simulink model "Hybrid_car_model"  (R2023a)
settings: Solver=VariableStepAuto  StartTime=0.0  StopTime=7200  MaxStep=0.05  RelTol=1e-3
values from neighbouring files (symbols this model uses):
  Af = 0.6    [a_Vehicle_Data.m]
  Cd = 0.5    [a_Vehicle_Data.m]
  eta_dt = 0.95    [a_Vehicle_Data.m]
  fR = 0.020    (= 0.02)    [a_Vehicle_Data.m]
  g = 9.81    [a_Vehicle_Data.m]
  gamma = 0    [a_Vehicle_Data.m]
  i_1 = 31/12    (= 2.58333333333)    [a_Vehicle_Data.m]
  i_2 = 25/13    (= 1.92307692308)    [a_Vehicle_Data.m]
  i_3 = 23/15    (= 1.53333333333)    [a_Vehicle_Data.m]
  i_4 = 24/19    (= 1.26315789474)    [a_Vehicle_Data.m]
  i_fin = 36/13    (= 2.76923076923)    [a_Vehicle_Data.m]
  i_prim = 56/22    (= 2.54545454545)    [a_Vehicle_Data.m]
  K_e = 1/54    (= 0.0185185185185)    [c_electric_motor_data.m]
  K_t = 0.15    [c_electric_motor_data.m]
  L_a = 23e-6    (= 2.3e-05)    [c_electric_motor_data.m]
  m = 250    [a_Vehicle_Data.m]
  R_a = 22.5e-3    (= 0.0225)    [c_electric_motor_data.m]
  r_dyn = 0.227    [a_Vehicle_Data.m]
  rho = 1.225    [a_Vehicle_Data.m]
  time_demand = [0;1;2;3;4;5;6;7;8;9;10;11;12;13;14;15;16;17;18;19;20;21;22;23;24;25;26;27;28;29;30;31;32;33;34;35;36;37;38;39;40;41;42;43;44;45;46;47;48;49;50;51;52;53;54;55;56;57;58;59;60;61;62;63;64;65;66;67;68;69;70;71;72;73;74;75;76;77;78;79;80;81;82;83;84;85;86;87;88;89;90;91;92;93;94;95;96;97;98;99;100;101;102;103;104;105;106;107;108;109;110;111;112;113;114;115;116;117;118;119;120;121;122;123;124;125;126;1 ...(+7496 chars)    [WLTP_data.m]
  velocity_demand = [0;0;0;0;0;0;0;0;0;0;0;0;0.200000000000000;1.70000000000000;5.40000000000000;9.90000000000000;13.1000000000000;16.9000000000000;21.7000000000000;26;27.5000000000000;28.1000000000000;28.3000000000000;28.8000000000000;29.1000000000000;30.8000000000000;31.9000000000000;34.1000000000000;36.6000000000000;39.1000000000000;41.3000000000000;42.5000000000000;43.3000000000000;43.9000000000000;44.40000000000 ...(+24040 chars)    [WLTP_data.m]
undefined symbols (not defined in the file or in its folder): Hydride, Metal, Nickel
libraries: spsCurrentMeasurementLib x2, spsBatteryLib x1, spsControlledCurrentSourceLib x1, spsDCMachineLib x1, sps_lib x1, slpidlib x1
settings Model: Creator=jens.lahr  LastModifiedBy=id306071
settings ModelReferenceCC: EnableRefExpFcnMdlSchedulingChecks=on

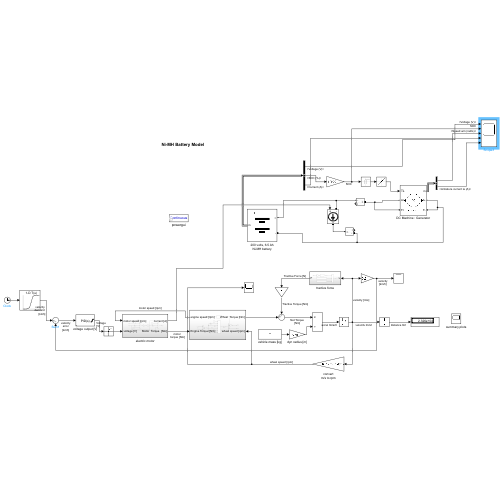
[thumbnail: Simulink's stored preview of the top-level diagram]
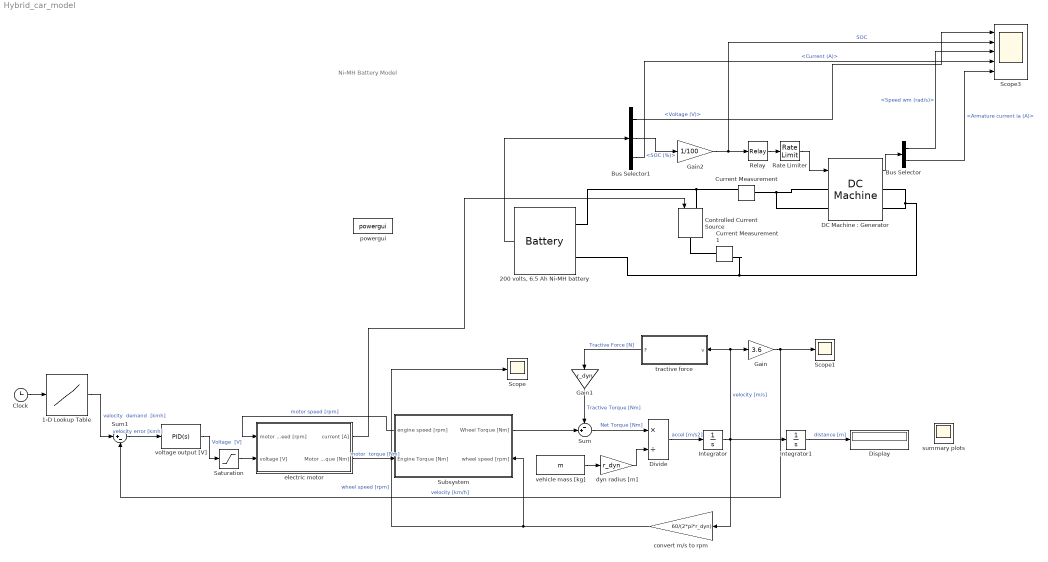
== system Hybrid_car_model ==
  note: Ni-MH Battery Model
  1-D Lookup Table : Lookup_n-D  NumberOfTableDimensions=1  BreakpointsForDimension1=time_demand  Table=velocity_demand  InternalRulePriority=Speed  RndMeth=Simplest
  "200 volts, 6.5 Ah Ni-MH battery " : spsBatteryLib/Battery  BatType=Nickel-Metal-Hydride  ShowTempParam=on  ThermalPreset=no  ShowAgeParam=off  NomV=200  NomQ=6.5  SOC=100  Batt_Tr=30  PresetModel=on  MaxQ=7  MinV=150  FullV=235.5932  Dis_rate=1.3  R=0.30769  Normal_OP=6.25  expZone="[216.9492           1.3]"  current=50  Units=Ampere-hour  Tci=20  NomT=25  T2=0  MaxQ2=2.208  FullV2=3.45  Normal_OP2=2.8  expZone2="[3.22        0.23]"  Rca=0.6  ti=1000  Dp=0  Neq0=0  Tsim=1e6  Ta1=25  Qeol=5.4*0.9  Reol=0.013333*1.2  Char_age=[2.3478, 3]  Dis_age=[2.3478, 10]  N1=1500  N2=10500  N3=1000  N4=1400  Ta2=45  N5=950
      settings: LibrarySourceBlock=electricdrivelib/Extra Sources/Battery
  Bus Selector : BusSelector  OutputSignals=Speed wm (rad/s),Armature current ia (A)
  Bus Selector1 : BusSelector  OutputSignals=Voltage (V),SOC (%),Current (A)
  Clock : Clock
  Controlled Current Source : spsControlledCurrentSourceLib/Controlled Current Source  Initialize=on  Source_Type=AC  Amplitude=0  Phase=0  Frequency=0  Measurements=None
  Current Measurement : spsCurrentMeasurementLib/Current Measurement  PhasorSimulation=off  OutputType=Complex  PSBequivalent=0
  Current Measurement1 : spsCurrentMeasurementLib/Current Measurement  PhasorSimulation=off  OutputType=Complex  PSBequivalent=0
  "DC Machine : Generator" : spsDCMachineLib/DC Machine  PresetModel=No  MechanicalLoad=Torque TL  FieldType=Wound  ShowDetailedParameters=on  MeasurementBus=off  RLa=[0.4832 0.006763]  RLf=[84.91 13.39]  Laf=0.7096  MachineConstant=Torque constant (N.m/A)  Ke=1.8  Kt=1.8  J=0.2053  Bm=0.007032  Tf=0  w0=0  Ifinit=0  TsPowergui=0  TsBlock=-1
  Display : Display
  Divide : Product  Inputs=*/
  Gain : Gain  Gain=3.6
  Gain1 : Gain  Gain=r_dyn
  Gain2 : Gain  Gain=1/100
  Integrator : Integrator  LimitOutput=on  LowerSaturationLimit=0
  Integrator1 : Integrator
  Rate Limiter : RateLimiter  RisingSlewLimit=100  FallingSlewLimit=-100
  Relay : Relay  OnSwitchValue=0.95  OffSwitchValue=0.2  OnOutputValue=0  OffOutputValue=-200
  Saturation : Saturate  UpperLimit=48  LowerLimit=0
  Scope : Scope
  Scope1 : Scope
  Scope3 : Scope  NumInputPorts=5
  Subsystem : Subsystem
      settings: PortSchema="{\"entries\":[{\"content\":{\"sides\":[{\"content\":{\"connectorIds\":[\"Out2\",\"In1\"]},\"type\":\"ConnectorPlacement.EquallySpacedRectSide\",\"uuid\":\"3db7130f-4414-4138-a483-769651bc2e03\"},{\"content\":{\"connectorIds\":[\"Out1\",\"In2\"],\"side\":\"RIGHT\"},\"type\":\"ConnectorPlacement.EquallySpacedRectSide\",\"uuid\":\"89f2a1b6-eda5-4fe5-b7f3-89dce8f6cd7c\"},{\"content\":{\"connectorIds\":[],\"side\":\"TOP\"},\"type\":\"ConnectorPlacement.EquallySpacedRectSide\",\"uuid\":\"e9ab6c0b-b883-402a-b7db-f259101e283a\"}]},\"type\":\"ConnectorPlacement.EquallySpacedConnector\",\"uuid\":\"5847757e-1c33-4a70-baac-f92835d7beeb\"}],\"packageUris\":[\"http://schema.mathworks.com/mf0/Connector/R2020b\"],\"version\":\"1.0\"}"
  Sum : Sum  Inputs=-+|
  Sum1 : Sum  Inputs=|+-
  convert m/s to rpm : Gain  Gain=60/(2*pi*r_dyn)
  dyn radius [m] : Gain  Gain=r_dyn
  electric motor : Subsystem
  powergui : sps_lib/powergui  SimulationMode=Continuous  SampleTime=0.001  frequency=60  Iterations=50  frequencyindice=0  Pbase=100e6  ErrMax=1e-4  UnitsV=kV  UnitsW=MW  buscounter=0  FunctionMessages=off  echomessages=off  EnableUseOfTLC=off  CurrentSourceSwitches=off  DisableSnubberDevices=off  DisableRonSwitches=off  DisableVfSwitches=off  DisplayEquations=off  AutomaticDiscreteSolvers=off  SolverType=Tustin  Interpol=off  ExternalGateDelay=off  methode=off  Ts=0  x0status=blocks  SPID=off  SwTol=0  HookPort=off  NonlinearTolerance=1e-4  nMaxIteration=100  ContinueOnMaxIteration=off  RestoreLinks=warning  ResistiveCurrentMeasurement=off  Frange=[0:2:500]  Ylog=off  Xlog=on  ShowGrid=off  save=off  variable=ZData  structure=0  ZoomFFT=on  StartTime=0.0  cycles=1  DisplayStyle=1  fundamental=60  FreqAxis=off  MaxFrequency=1000  frequencyindicesteady=1  RmsSteady=1  display=off
  summary plots : Scope
      settings: Floating=on
  tractive force : Subsystem
  vehicle mass [kg] : Constant  Value=m
  voltage output [V] : slpidlib/PID Controller  Controller=PID  Form=Parallel  TimeDomain=Continuous-time  UseExternalTs=off  SampleTime=-1  IntegratorMethod=Forward Euler  FilterMethod=Forward Euler  ControllerParametersSource=internal  P=23.06  I=0.5  UseKiTs=off  D=0  N=100  UseFilter=on  TunerSelectOption=Transfer Function Based (PID Tuner App)  InitialConditionSource=internal  InitialConditionForIntegrator=0  InitialConditionForFilter=0  DifferentiatorICPrevScaledInput=0  ExternalReset=none  TrackingMode=off  Kt=1  LimitOutput=on  SatLimitsSource=internal  UpperSaturationLimit=48  LowerSaturationLimit=0  LinearizeAsGain=on  AntiWindupMode=none  Kb=1  LimitIntegrator=off  UpperIntegratorSaturationLimit=inf  LowerIntegratorSaturationLimit=-inf  POutMin=[]  POutMax=[]  IOutMin=[]  IOutMax=[]  DOutMin=[]  DOutMax=[]  NOutMin=[]  NOutMax=[]  SumOutMin=[]  SumOutMax=[]  SaturationOutMin=[]  SaturationOutMax=[]  PParamMin=[]  PParamMax=[]  IParamMin=[]  IParamMax=[]  DParamMin=[]  DParamMax=[]  NParamMin=[]  NParamMax=[]  KbParamMin=[]  KbParamMax=[]  KtParamMin=[]  KtParamMax=[]  KbOutMin=[]  KbOutMax=[]  KtOutMin=[]  KtOutMax=[]  IntegratorOutMin=[]  IntegratorOutMax=[]  FilterOutMin=[]  FilterOutMax=[]  SumI1OutMin=[]  SumI1OutMax=[]  SumI2OutMin=[]  SumI2OutMax=[]  SumI3OutMin=[]  SumI3OutMax=[]  SumI4OutMin=[]  SumI4OutMax=[]  SumDOutMin=[]  SumDOutMax=[]  DifferentiatorOutMin=[]  DifferentiatorOutMax=[]  FilterDiffOutCoefMin=[]  FilterDiffOutCoefMax=[]  ReciprocalOutMin=[]  ReciprocalOutMax=[]  SumDenOutMin=[]  SumDenOutMax=[]  SumNumOutMin=[]  SumNumOutMax=[]  DivideOutMin=[]  DivideOutMax=[]  UdiffTsProdOutMin=[]  UdiffTsProdOutMax=[]  NTsProdOutMin=[]  NTsProdOutMax=[]  UintegralTsProdOutMin=[]  UintegralTsProdOutMax=[]  UngainTsProdOutMin=[]  UngainTsProdOutMax=[]  ClampingZeroOutDataTypeStr=Inherit: Inherit via back propagation  ClampingZeroOutMin=[]  ClampingZeroOutMax=[]  FilterDenConstantOutDataTypeStr=Inherit: Inherit via back propagation  FilterDenConstantOutMin=[]  FilterDenConstantOutMax=[]  PCopyOutDataTypeStr=Inherit: Inherit via back propagation  PCopyOutMin=[]  PCopyOutMax=[]  NCopyOutDataTypeStr=Inherit: Inherit via back propagation  NCopyOutMin=[]  NCopyOutMax=[]  IntegratorContinuousStateAttributes=''  IntegratorStateMustResolveToSignalObject=off  IntegratorRTWStateStorageClass=Auto  FilterContinuousStateAttributes=''  FilterStateMustResolveToSignalObject=off  FilterRTWStateStorageClass=Auto  ParallelPVariant=InternalParameters  IdealPVariant=Disabled  IVariant=InternalParameters  DVariant=InternalParameters  IntegratorVariant=Continuous  SatVariant=Enabled  AWVariant=Passthrough  PCopyVariant=Disabled  TRVariant=Disabled  FdbkBlocksVariant=Forward  IdealPFdbkVariant=Disabled  SatFdbkVariant=Disabled  DerivativeFilterVariant=ContFilter  NVariant=InternalParameters  NCopyVariant=Disabled  FilterICVariant=InternalICsFilter  IntegratorICVariant=InternalICs  ExternalResetVariant=Disabled  TRSumVariant=Passthrough  SumFdbkVariant=Disabled  SumVariant=Sum_PID  TsampFilterVariant=InternalTs  TsampNgainVariant=Passthrough  TsampIntegralVariant=Disabled_SignalSpec  ExternalSaturationOutDataTypeStr=Inherit: Same as second input
  wires:
  Divide/1 -> Integrator/1  "accel [m/s2]"
  Integrator/1 -> Gain/1, tractive force/1(v), Integrator1/1, convert m/s to rpm/1  "velocity [m/s]"
  Integrator1/1 -> Display/1  "distance [m]"
  vehicle mass [kg]/1 -> dyn radius [m]/1
  dyn radius [m]/1 -> Divide/2
  Sum/1 -> Divide/1  "Net Torque [Nm]"
  tractive force/1(F) -> Gain1/1  "Tractive Force [N]"
  Gain1/1 -> Sum/1  "Tractive Torque [Nm]"
  convert m/s to rpm/1 -> Scope/1, Subsystem/2(wheel speed [rpm])  "wheel speed [rpm]"
  Subsystem/1(Wheel Torque [Nm]) -> Sum/2
  Gain/1 -> Scope1/1, Sum1/2  "velocity [km/h]"
  Sum1/1 -> voltage output [V]/1  "velocity error [kmh]"
  1-D Lookup Table/1 -> Sum1/1  "velocity  demand  [kmh]"
  Clock/1 -> 1-D Lookup Table/1
  electric motor/2(Motor Torque [Nm]) -> Subsystem/1(Engine Torque [Nm])  "motor  torque [Nm]"
  Subsystem/2(engine speed [rpm]) -> electric motor/1(motor speed [rpm])  "motor speed [rpm]"
  Bus Selector1/3 -> Scope3/4  "<Current (A)>"
  "DC Machine : Generator"/1 -> Bus Selector/1
  Rate Limiter/1 -> "DC Machine : Generator"/1
  "200 volts, 6.5 Ah Ni-MH battery "/1 -> Bus Selector1/1
  Bus Selector/1 -> Scope3/3  "<Speed wm (rad/s)>"
  Bus Selector1/1 -> Scope3/1  "<Voltage (V)>"
  Bus Selector1/2 -> Gain2/1  "<SOC (%)>"
  Gain2/1 -> Relay/1, Scope3/2  "SOC"
  Relay/1 -> Rate Limiter/1
  Bus Selector/2 -> Scope3/5  "<Armature current ia (A)>"
  electric motor/1(current [A]) -> Controlled Current Source/1
  Saturation/1 -> electric motor/2(voltage [V])
  voltage output [V]/1 -> Saturation/1  "Voltage  [V]"
  connections:
  Controlled Current Source/LConn1 -- "200 volts, 6.5 Ah Ni-MH battery "/LConn1 -- Current Measurement/RConn1
  Current Measurement/LConn1 -- "DC Machine : Generator"/LConn2 -- "DC Machine : Generator"/LConn1
  "DC Machine : Generator"/RConn1 -- Current Measurement1/RConn1 -- "200 volts, 6.5 Ah Ni-MH battery "/LConn2 -- "DC Machine : Generator"/RConn2
  Current Measurement1/LConn1 -- Controlled Current Source/RConn1

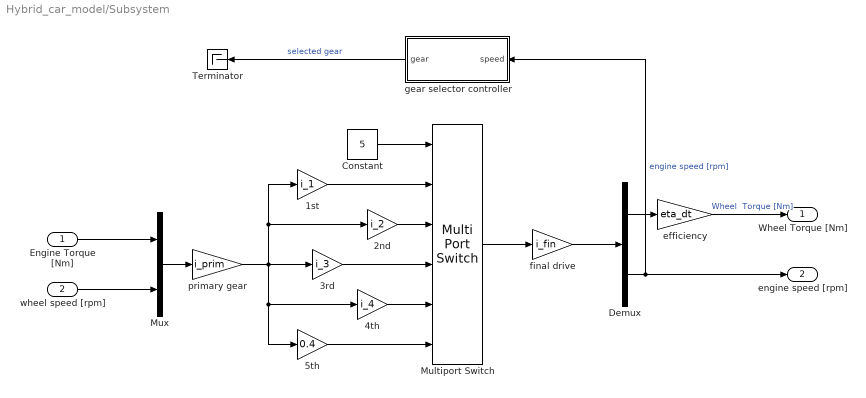
== system Hybrid_car_model/Subsystem ==
  Engine Torque [Nm] : Inport
  wheel speed [rpm] : Inport  Port=2
  1st : Gain  Gain=i_1
  2nd : Gain  Gain=i_2
  3rd : Gain  Gain=i_3
  4th : Gain  Gain=i_4
  5th : Gain  Gain=0.4
  Constant : Constant  Value=5
  Demux : Demux  Outputs=2
  Multiport Switch : MultiPortSwitch  Inputs=5  SaturateOnIntegerOverflow=off  InputSameDT=off
  Mux : Mux  Inputs=2
  Terminator : Terminator
  efficiency : Gain  Gain=eta_dt
  final drive : Gain  Gain=i_fin
  gear selector controller : Subsystem
  primary gear : Gain  Gain=i_prim
  Wheel Torque [Nm] : Outport
  engine speed [rpm] : Outport  Port=2
  wires:
  efficiency/1 -> Wheel Torque [Nm]/1  "Wheel  Torque [Nm]"
  Demux/2 -> gear selector controller/1(speed), engine speed [rpm]/1  "engine speed [rpm]"
  Engine Torque [Nm]/1 -> Mux/1
  wheel speed [rpm]/1 -> Mux/2
  primary gear/1 -> 1st/1, 2nd/1, 5th/1, 4th/1, 3rd/1
  1st/1 -> Multiport Switch/2
  Multiport Switch/1 -> final drive/1
  final drive/1 -> Demux/1
  2nd/1 -> Multiport Switch/3
  3rd/1 -> Multiport Switch/4
  4th/1 -> Multiport Switch/5
  5th/1 -> Multiport Switch/6
  Mux/1 -> primary gear/1
  Demux/1 -> efficiency/1
  gear selector controller/1(gear) -> Terminator/1  "selected gear"
  Constant/1 -> Multiport Switch/1

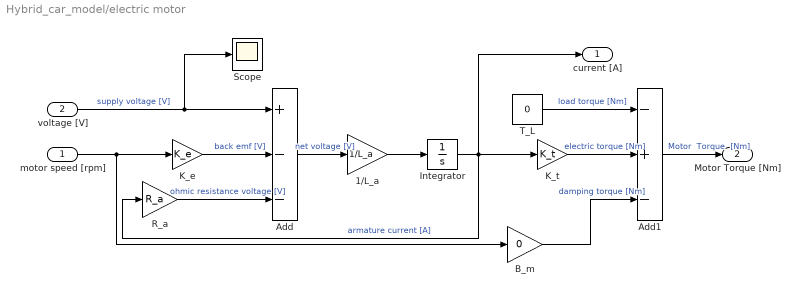
== system Hybrid_car_model/electric motor ==
  motor speed [rpm] : Inport
  voltage [V] : Inport  Port=2
  1/L_a : Gain  Gain=1/L_a
  Add : Sum  Inputs=+--
  Add1 : Sum  Inputs=-+-
  B_m : Gain  Gain=0
  Integrator : Integrator  LimitOutput=on  UpperSaturationLimit=400  LowerSaturationLimit=-400
  K_e : Gain  Gain=K_e
  K_t : Gain  Gain=K_t
  R_a : Gain  Gain=R_a
  Scope : Scope
  T_L : Constant  Value=0
  current [A] : Outport
  Motor Torque [Nm] : Outport  Port=2
  wires:
  Add1/1 -> Motor Torque [Nm]/1  "Motor  Torque  [Nm]"
  K_t/1 -> Add1/2  "electric torque [Nm]"
  voltage [V]/1 -> Scope/1, Add/1  "supply voltage [V]"
  B_m/1 -> Add1/3  "damping torque [Nm]"
  R_a/1 -> Add/3  "ohmic resistance voltage [V]"
  1/L_a/1 -> Integrator/1
  K_e/1 -> Add/2  "back emf [V]"
  Add/1 -> 1/L_a/1  "net voltage [V]"
  Integrator/1 -> current [A]/1, K_t/1, R_a/1  "armature current [A]"
  T_L/1 -> Add1/1  "load torque [Nm]"
  motor speed [rpm]/1 -> B_m/1, K_e/1

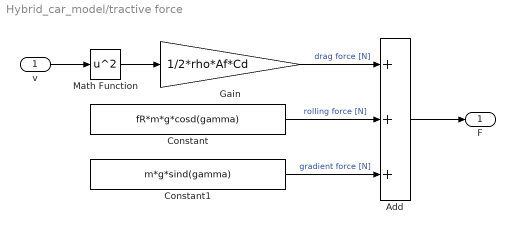
== system Hybrid_car_model/tractive force ==
  v : Inport
  Add : Sum  Inputs=+++
  Constant : Constant  Value=fR*m*g*cosd(gamma)
  Constant1 : Constant  Value=m*g*sind(gamma)
  Gain : Gain  Gain=1/2*rho*Af*Cd
  Math Function : Math  Operator=square
  F : Outport
  wires:
  v/1 -> Math Function/1
  Math Function/1 -> Gain/1
  Gain/1 -> Add/1  "drag force [N]"
  Add/1 -> F/1
  Constant/1 -> Add/2  "rolling force [N]"
  Constant1/1 -> Add/3  "gradient force [N]"

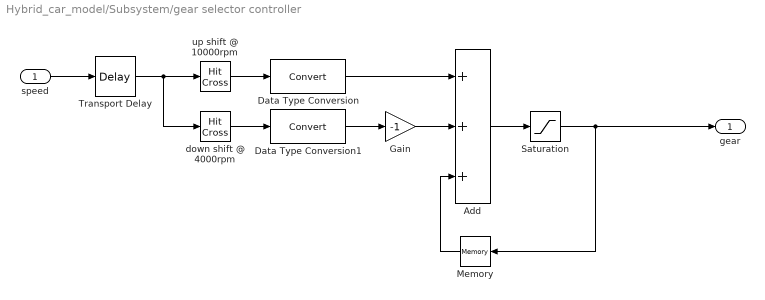
== system Hybrid_car_model/Subsystem/gear selector controller ==
  speed : Inport
  Add : Sum  Inputs=+++
  Data Type Conversion : DataTypeConversion  SaturateOnIntegerOverflow=off  RndMeth=Floor
  Data Type Conversion1 : DataTypeConversion  SaturateOnIntegerOverflow=off  RndMeth=Floor
  Gain : Gain  Gain=-1
  Memory : Memory  InitialCondition=1
  Saturation : Saturate  UpperLimit=5  LowerLimit=1
  Transport Delay : TransportDelay  DelayTime=0.01
  down shift @ 4000rpm : HitCross  HitCrossingOffset=2000  HitCrossingDirection=falling
  up shift @ 10000rpm : HitCross  HitCrossingOffset=5000  HitCrossingDirection=rising
  gear : Outport
  wires:
  speed/1 -> Transport Delay/1
  up shift @ 10000rpm/1 -> Data Type Conversion/1
  Data Type Conversion/1 -> Add/1
  down shift @ 4000rpm/1 -> Data Type Conversion1/1
  Data Type Conversion1/1 -> Gain/1
  Transport Delay/1 -> down shift @ 4000rpm/1, up shift @ 10000rpm/1
  Gain/1 -> Add/2
  Add/1 -> Saturation/1
  Saturation/1 -> Memory/1, gear/1
  Memory/1 -> Add/3
